simulink model "Position_System_control101"  (R2023a)
settings: Solver=ode45  StartTime=1.0  StopTime=stoptime  RelTol=1e-4  EnableMultiTasking=on
values from neighbouring files (symbols this model uses):
  C = 6000    [simulink_openloop_model_control101_script.m]    (also in simulink_openloop_modelb_control101_script.m; simulink_openloop_modelc_control101_script.m = 2000; simulink_openloop_modeld_control101_script.m = 1000)
undefined symbols (not defined in the file or in its folder): d, km, ks, P, R
settings Model: Creator=co1gp  LastModifiedBy=Anthony Rossiter
settings SolverCC: AlgebraicLoopSolver=TrustRegion
settings DataIOCC: SaveFinalState=on  SaveFormat=Array  SignalLoggingSaveFormat=ModelDataLogs  SaveState=on  ReturnWorkspaceOutputs=off
settings OptimizationCC: BooleanDataType=off  ExpressionDepthLimit=2147483647  LifeSpan=inf
settings DebuggingCC: SaveWithParameterizedLinksMsg=none  UnderspecifiedInitializationDetection=Classic  MergeDetectMultiDrivingBlocksExec=none  SignalResolutionControl=TryResolveAllWithWarning  InheritedTsInSrcMsg=none  MultiTaskDSMMsg=warning  MultiTaskCondExecSysMsg=none  FcnCallInpInsideContextMsg=warning  UnconnectedInputMsg=warning  UnconnectedOutputMsg=warning  UnconnectedLineMsg=warning  StateNameClashWarn=warning  SFUnexpectedBacktrackingDiag=warning  SFNoUnconditionalDefaultTransitionDiag=warning  SFExecutionAtInitializationDiag=none  ArithmeticOperatorsInVariantConditions=warning
settings HardwareCC: ProdBitPerPointer=32  ProdBitPerSizeT=32  ProdBitPerPtrDiffT=32  ProdLargestAtomicFloat=None  ProdIntDivRoundTo=Undefined  ProdEndianess=Unspecified  ProdWordSize=32  ProdHWDeviceType=32-bit Generic  TargetUnknown=on
settings ModelReferenceCC: EnableRefExpFcnMdlSchedulingChecks=on  PropagateSignalLabelsOutOfModel=off
settings SFSimCC: SimUseLocalCustomCode=off  CustomCodeUndefinedFunction=UseInterfaceOnly
settings RTWCC: RTWUseLocalCustomCode=off  DLArmComputeVersion=19.05
settings CodeAppCC: StateflowObjectComments=on
settings GRTTargetCC: TargetLangStandard=C89/C90 (ANSI)  CombineOutputUpdateFcns=off  GRTInterface=on
settings ConfigComp: CovMetricSettings=dw  CovSaveCumulativeToWorkspaceVar=on  CovSaveSingleToWorkspaceVar=on

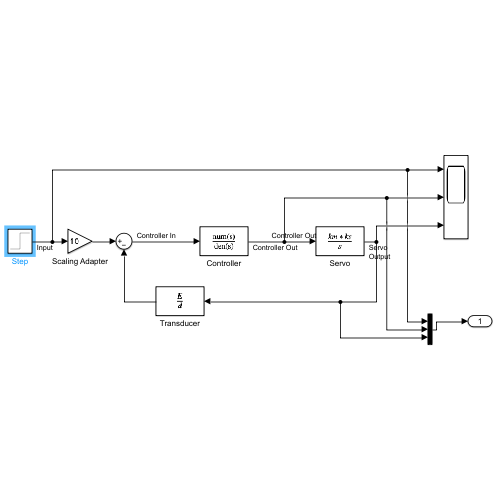
[thumbnail: Simulink's stored preview of the top-level diagram]
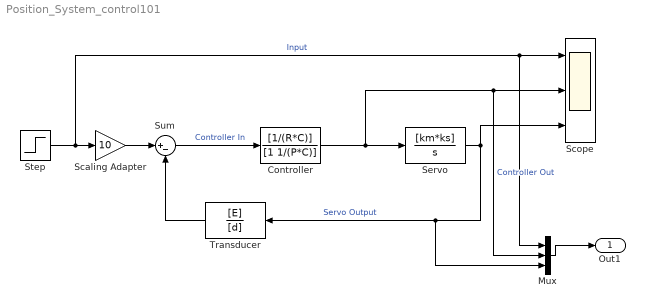
== system Position_System_control101 ==
  Controller : TransferFcn  Numerator=[1/(R*C)]  Denominator=[1 1/(P*C)]
  Mux : Mux  Inputs=3
  Scaling Adapter : Gain  Gain=10  SaturateOnIntegerOverflow=on  OutDataTypeStr=Inherit: Same as input  ParamDataTypeStr=Inherit: Same as input
  Scope : Scope  NumInputPorts=3
  Servo : TransferFcn  Numerator=[km*ks]  Denominator=[1 0]
  Step : Step  After=1.3
  Sum : Sum  Inputs=|+-  InputSameDT=on  SaturateOnIntegerOverflow=on  OutDataTypeStr=Inherit: Same as first input
  Transducer : TransferFcn  Numerator=[E]  Denominator=[d]
  Out1 : Outport
  wires:
  Step/1 -> Scaling Adapter/1, Mux/1, Scope/1  "Input"
  Scaling Adapter/1 -> Sum/1
  Sum/1 -> Controller/1  "Controller In"
  Servo/1 -> Mux/3, Transducer/1, Scope/3  "Servo Output"
  Transducer/1 -> Sum/2
  Controller/1 -> Scope/2, Mux/2, Servo/1  "Controller Out"
  Mux/1 -> Out1/1
